simulink model "vmr_rwd_fix_leftarm"  (R2015a)
settings: Solver=ode4  SolverMode=MultiTasking  StartTime=0.0  StopTime=inf  FixedStep=BKIN_STEP_TIME  RelTol=1e-3
StartFcn:
  |  warndlg('Dexterit-E models cannot run under simulation. Please compile your model and run it from within Dexterit-E.');set_param(bdroot,'SimulationCommand','stop')
model workspace (MAT data in the model file):
  BKIN_STEP_TIME = 0.00025
  col_x = 1
  col_y = 2
  E_TARGET_ON = 3
  LOGICAL_RADIUS = 4
  START_TARGET_COL = 1
  END_TARGET_COL = 2
  ROTATION_CENTER = 3
  MAXREACHTIME_COL = 5
  ROTATION_TYPE = 7
  ROTATION = 8
  DELAY_POSTTRIAL_COL = 6
  E_STAY_CENTER = 2
  VISUAL_RADIUS = 3
  COLOR = 5
  K_SCORETEXT_ROW = 1
  LABEL_HEIGHT = 8
  HITCOLOR = 6
  E_HIT_TARGET = 5
  E_MISS_TARGET = 9
  K_REWARD_VAL = 2
  K_TONE_HIT_DURATION = 4
  K_TONE_HIT_FREQUENCY = 5
  K_VIS_RAD = 6
  E_REWARD = 6
  WAIT_AT_START_COL = 4
  LABEL = 7
  K_RETURN_RING_ROW = 7
  STROKE_WIDTH = 9
  STROKE_COLOR = 10
  K_SCORE_TIME = 8
  HAND_VIS_COL = 9
  CLAMP_COL = 10
  DO_REWARD_COL = 11
  K_TONE_NEUTRAL_DURATION = 10
  K_TONE_NEUTRAL_FREQUENCY = 11
  E_NEUTRAL_FDBK = 10
  E_SHOW_SCORE = 17
  DISPLAY_TRIAL_COL = 12
  K_INSTRUCT_TIME = 9
  E_SHOW_INSTRUCT = 18
  INSTRUCT_PAUSE_BTN = 2
  K_LEFTHAND_TGT = 12
  K_ROBOT_RAMP_TIME = 14
  K_ROBOT_MOVE_TIME = 15
  K_FIX_LEFTHAND = 13
  BKIN_KINEMATIC_FRAME_SIZE = 400
  E_NO_EVENT = 0
  K_UNUSED = 3
  ROTATED_COLOR = 11
undefined symbols (not defined in the file or in its folder): slselsubs
libraries: Video x9, slrtlib x7, General x3, KINARM_general x2, KINARM_loads x2, simulink x1, xpcnilib x1
(part 2 of 2)

== stateflow chart vmr_rwd_fix_leftarm/Trial_Control ==
  settings: sampleTime=0.001
  state MoveHandAway/
    robot_enable_controller = 1;
    tickCount = TaskwideParams[K_ROBOT_RAMP_TIME];
    tickCount += TaskwideParams[K_ROBOT_MOVE_TIME];
  state Initialize/
    // Turn off both targets, set hand_feedback on
    targetA_state=0;
    targetB_state=0;
    reward_state = 0;
    score = 0;
    rotation_on = 0;
    handvis_state = 1;
    reward_type = 0;
    instruct_num = 0;
    fdbk_text = 0;
    robot_enable_controller = 0;
  state InitStartTarget/
    // Turn on first target, wait until hand-is-in-target
    targetA_row = Trial_Protocol[START_TARGET_COL];
    targetA_state=1;
    handvis_state = 1;
    rotation_on = 0;
  state Main_Trial
    state StartTargetOn/
      // Turn on first target, wait until hand-is-in-target
      targetA_row = Trial_Protocol[START_TARGET_COL];
      targetA_state=1;
      handvis_state = 1;
      rotation_on = 0;
      logging_enable = 1;
      reward_type = Trial_Protocol[DO_REWARD_COL];
      tone = 0;
    state StayAtFirstTarget/
      // change the first target state (e.g. colour), log an event, wait for specified period of time.  Hand must STAY in target for specified time.
      event_code=E_STAY_CENTER;
      tickCount =Trial_Protocol[WAIT_AT_START_COL];
    state WaitForSound/
    state Show2ndTarget/
      // Turn on second target, log an event, wait until hand-is-in-target or wait for specified delay
      event_code=E_TARGET_ON;
      targetB_row = Trial_Protocol[END_TARGET_COL];
      targetB_state= 1 + 2*double(rotation_on > 0 || do_clamp > 0);
      tickCount =Trial_Protocol[MAXREACHTIME_COL];
      tick = 0;
      dist  = TargetDistance[START_TARGET_COL][END_TARGET_COL];
      during:
      on e_clk: tick++;
    state Hit2ndTarget/
      // change the 2nd target's state, log an event, wait for the rest of the trial to end
      event_code=E_HIT_TARGET;
    state Miss2ndTarget/
      //if hand exceeds target ring, trial is over
      event_code = E_MISS_TARGET;
      targetB_state = 0;
      reward_state = 0;
      handvis_state = 0;
      rotation_on = 0;
      during:
      on e_clk: tick++;
    state TooSlowState/
      fdbk_text = -1;  //"too slow"
      targetA_state = 2;
      rotation_on = 0;
      handvis_state = 0;
      //fdbk_text = 1; //"too fast"
    state DoReward/
      event_code = E_REWARD;
      targetB_state=2;
      reward_state=1;
      reward = TaskwideParams[K_REWARD_VAL];
      score += reward;
      fdbk_text = 0;
      tone = 1;
      handvis_state = 0;
      rotation_on = 0;
      during:
      on e_clk: tick++;
    state NeutralReward/
      event_code = E_NEUTRAL_FDBK;
      //do this state if we are in a clamped or aftereffect trial to indicate end of trial
      handvis_state = 0;
      reward_state = 0;
      fdbk_text = 0;
      rotation_on = 0;
      tone = 2;
      //do nothing
      during:
      on e_clk: tick++;
    state NoReward/
      handvis_state = 0;
      fdbk_text = 0;
      rotation_on = 0;
      //do nothing
      during:
      on e_clk: tick++;
    state EndOfTrial/
      // Wait for a specified period of time,
      targetB_state = 0;
      handvis_state = 2;
      do_clamp = 0;
      rotation_on = 0;
    StartTargetOn -> StayAtFirstTarget : [HandInTarget[targetA_row]==1]
    StayAtFirstTarget -> StartTargetOn [order 2] : [HandInTarget[targetA_row]==0]
    StayAtFirstTarget -> WaitForSound [order 1] : after(tickCount, e_clk)/
        | rotation_on = Trial_Protocol[ROTATION_TYPE];
        | handvis_state = Trial_Protocol[HAND_VIS_COL];
        | do_clamp = Trial_Protocol[CLAMP_COL];
        | e_ApplyNewRotation
        | // apply the new rotation amount now (i.e. wait until hand is in the start target so that
        | // the hand feedback doesn't jump when a new rotation is applied)
    WaitForSound -> Show2ndTarget : [soundON == 0]
    Show2ndTarget -> TooSlowState [order 1] : [tick >= tickCount]
        | //max trial duration specified by tickCount
    Show2ndTarget -> Miss2ndTarget [order 2] : [DistFromTarget[targetA_row] >= dist]
    Show2ndTarget -> Hit2ndTarget [order 3] : [HandInTarget[targetB_row]==1]
    Hit2ndTarget -> DoReward [order 3] : [reward_type == 1]
        | //do the reward
    Hit2ndTarget -> NoReward [order 2] : [reward_type == 0]
        | //no reward
    Hit2ndTarget -> NeutralReward [order 1] : [reward_type == 2]
        | //neutral feedback tone
    Miss2ndTarget -> NeutralReward [order 2] : [reward_type == 2]
        | //neutral feedback tone
    TooSlowState -> EndOfTrial
    Miss2ndTarget -> EndOfTrial [order 1] : //after(tickCount, e_clk)
        | [reward_type != 2 && tick >= tickCount]
    NoReward -> EndOfTrial : //after(tickCount, e_clk)
        | [tick >= tickCount]
    NeutralReward -> EndOfTrial : //after(tickCount, e_clk)
        | [tick >= tickCount]
    DoReward -> EndOfTrial : //after(tickCount, e_clk)
        | [tick >= tickCount]
  state Ending/
    //end the special "show score" state
    e_Trial_End;
  state EndInstructPause/
    instruct_num = 0;
    handvis_state = 1;
    targetA_state = 1;
    tickCount = 800;
  state ReturnToStart1/
    targetA_state=1;
    handvis_state = 1;
    reward_state = 0;
    instruct_num = 0;
  state InstructWaitState/
    //"pause" here until the button has been clicked
  state ShowScoreState/
    event_code = E_SHOW_SCORE;
    targetA_state = 0;
    targetB_state = 0;
    handvis_state = 1;
    reward_state = 2;
    tickCount = TaskwideParams[K_SCORE_TIME];
  state ShowInstructState/
    event_code = E_SHOW_INSTRUCT;
    targetA_state = 0;
    targetB_state = 0;
    handvis_state = 0;
    reward_state = 0;
    instruct_num = Trial_Protocol[DISPLAY_TRIAL_COL];
    tickCount = TaskwideParams[K_INSTRUCT_TIME];
  state Inter_Trial_State/
    // send e_Trial_End event
    e_Trial_End;
    // turn off both targets
    // stop data logging
    event_code=0;
    targetA_state=1; //don't shut off
    targetB_state=0;
    //logging_enable = 0;
    rotation_on = 0;
    fdbk_text = 0;
  state ReturnToStart/
    //targetA_state=1;
    handvis_state = 1;
    reward_state = 0;
    instruct_num = 0;
    tickCount =50;
  state Inter_Trial_Hold/
    //temporarily hold here until the hand gets close to the target
    tickCount = Trial_Protocol[DELAY_POSTTRIAL_COL];
  InitStartTarget -> MoveHandAway [order 1] : [HandInTarget[targetA_row]==1 && TaskwideParams[K_FIX_LEFTHAND] == 1]
      | //if we want to hold the left hand, enable the robot
  (default) -> Initialize
  MoveHandAway -> (junction 112) : after(tickCount,e_clk)
  Initialize -> InitStartTarget : after(1,e_clk)
  InitStartTarget -> (junction 112) [order 2] : [TaskwideParams[K_FIX_LEFTHAND] ~= 1]
      | //if we aren't going to enable the robot
  (junction 112) -> StartTargetOn [order 1] : [Trial_Protocol[DISPLAY_TRIAL_COL] <= 0]
      | //the first trial is a target trial
  (junction 112) -> ShowInstructState [order 2] : //the first trial is an instruction trial
      | [Trial_Protocol[DISPLAY_TRIAL_COL] > 0]
  ReturnToStart1 -> StartTargetOn : after(1, e_clk)
  Ending -> EndInstructPause : after(1,e_clk)/
      | //continue if a regular trial comes after!
  InstructWaitState -> Ending : e_cntl_btn/
      | event_code = 22;
  ShowScoreState -> Ending : after(tickCount,e_clk)
  EndInstructPause -> ReturnToStart1 : after(tickCount,e_clk)
  ShowInstructState -> InstructWaitState
  (junction 74) -> ReturnToStart1 [order 1] : [Trial_Protocol[DISPLAY_TRIAL_COL] == 0]
  (junction 74) -> ShowScoreState [order 2] : [Trial_Protocol[DISPLAY_TRIAL_COL] == -1]
  (junction 74) -> ShowInstructState [order 3] : [Trial_Protocol[DISPLAY_TRIAL_COL] > 0]
  Inter_Trial_State -> (junction 74) : after(1,e_clk)
  Main_Trial -> Inter_Trial_State : e_ExitTrialNow/
      | // if e_ExitTrialNow event occurs...
      | tickCount=1;
  ReturnToStart -> Inter_Trial_State : after(tickCount,e_clk)
  Inter_Trial_Hold -> ReturnToStart : [ DistFromTarget[targetA_row] <= TaskwideParams[K_VIS_RAD] && after(tickCount,e_clk) ]
      | //if the hand is close to the start, turn vision of the hand back on
  EndOfTrial -> Inter_Trial_Hold
  data: logging_enable output boolean; event_code output double; Trial_Protocol input double; targetA_row output [1..32]; targetA_state output double; targetB_row output double; targetB_state output double; tickCount local double; reward_state output double; score output int32; reward output int32; fdbk_text output int32; instruct_num output double; tone output double; TaskwideParams input double; HandInTarget input double; DistFromTarget input double; TargetDistance input double; reward_type local double; rotation_on output double; dist local double; tick local double; handvis_state output double; do_clamp output double; E_SHOW_INSTRUCT parameter; robot_enable_controller output boolean; soundON input double size=1
  data targetA_row settings: description=index of the row currently being used in the TargetTable
  events: e_ApplyNewRotation output EITHER_EDGE_EVENT; e_clk input RISING_EDGE_EVENT; e_ExitTrialNow input EITHER_EDGE_EVENT; e_Trial_End output EITHER_EDGE_EVENT; e_cntl_btn input EITHER_EDGE_EVENT

== matlab function vmr_rwd_fix_leftarm/Visual_Rotation/Triggered Subsystem/Embedded MATLAB Function ==
  settings: fimath=|
      | fimath(...
      | 'RoundMode', 'floor',...
      | 'OverflowMode', 'wrap',...
      | 'ProductMode', 'KeepLSB', 'ProductWordLength', 32,...
      | 'SumMode', 'KeepLSB', 'SumWordLength', 32,...
      | 'CastBeforeSum', false)
  data: rotate_on input; rotation output; Trial_Protocol input
function rotation   = Calculate_Desired_Rotation(rotate_on,Trial_Protocol)
% This block supports an embeddable subset of the MATLAB language.
% See the help menu for details. 

%This block was modified by IEB, Sept 24, 2008
%It updates the desired amount of rotation

% NOTE ALL ROTATIONS ARE CURRENTLY IN DEGREES IN THE FUNCTION

% create a persistent variable to remember the rotation amount from one time-step to the next
persistent rotation_memory

if isempty(rotation_memory),            rotation_memory = 0;										end

% where to look in the TP table for these parameters
rotate_type_COL = 7;
rotation_amount_COL = 8;

rotate_type = Trial_Protocol(rotate_type_COL);
rotation_amount = Trial_Protocol(rotation_amount_COL);

if rotate_type == 0 || rotate_on == 0
	%set the rotation = 0
	rotation = 0;
elseif rotate_type ==1 && rotate_on > 0
	%set the rotation = specified amount
	rotation = rotation_amount;
elseif rotate_type == 2 && rotate_on > 0
	%set the rotation to change by specified amount
	rotation = rotation_memory + rotation_amount;
else
	%do nothing
	rotation = rotation_memory;
end

% save the rotation amount for the next time-step
rotation_memory = rotation;

== matlab function vmr_rwd_fix_leftarm/Visual_Rotation/Embedded MATLAB Function ==
  settings: fimath=|
      | fimath(...
      | 'RoundMode', 'floor',...
      | 'OverflowMode', 'wrap',...
      | 'ProductMode', 'KeepLSB', 'ProductWordLength', 32,...
      | 'SumMode', 'KeepLSB', 'SumWordLength', 32,...
      | 'CastBeforeSum', false)
  data: CursorPos output; rotation input; TGT_VCODES_IN input; VCODES_IN input; feedback_state input; VCODES output
function [CursorPos,VCODES]  = Rotation(rotation, TGT_VCODES_IN,VCODES_IN,feedback_state) %Trial_Protocol, Target_Table,
% This block supports an embeddable subset of the MATLAB language.
% See the help menu for details. 

%This block was modified by IEB, Sept 24, 2008
%It rotates the cursor position around a location specified as a target in the Trial_Protocol.

% VCODEs are length VCODE_LENGTH.
% All dimensions are units of (m).
% VCODE index definition: 1-5 as the same for all target types
% 1 - Target type
%		1=circle
%		2=ellipse
%       3=rectangle
%		4=line
%       5=triangle
%		6 and higher - not implemented yet
% 2 - status
%		0=off
%		1=on
% 3 - x position (m)
% 4 - y position (m)

% column in target table to find the target to rotation about
rotation_center_COL = 3;

%rotation_center_target = Trial_Protocol(rotation_center_COL);
%x_center = Target_Table(rotation_center_target, 1) * 0.01;		%convert to meters
%y_center = Target_Table(rotation_center_target, 2) * 0.01;		%convert to meters
x_center = TGT_VCODES_IN(3);
y_center = TGT_VCODES_IN(4);

rotation = rotation*pi/180;		%convert desired rotation from degrees to radians

VCODES = VCODES_IN;
CursorPos = VCODES(1:2,3:4);
T = [x_center, y_center; x_center, y_center];                       %translation matrix
R = [cos(rotation) -sin(rotation); sin(rotation) cos(rotation)];	%rotation matrix

CursorPos = CursorPos - T;				%translate
CursorPos = (R*CursorPos')';			%rotate
CursorPos = CursorPos + T;				%re-translate

VCODES(1:2,3:4) = CursorPos;			%apply updated positions back into the VCODEs		

VCODES(1:2,1) = VCODES(1:2,1) & feedback_state;

== matlab function vmr_rwd_fix_leftarm/KINARM_HandFeedbackInTarget/Embedded MATLAB InsideTarget ==
  settings: fimath=|
      | fimath(...
      | 'RoundMode', 'floor',...
      | 'OverflowMode', 'wrap',...
      | 'ProductMode', 'KeepLSB', 'ProductWordLength', 32,...
      | 'SumMode', 'KeepLSB', 'SumWordLength', 32,...
      | 'CastBeforeSum', false)
  data: handpos input size=2; target_type input; attribcol input; num_targets input; intarget output; Target_Table input
function intarget = FIsInsideTarget(handpos, target_type, attribcol, num_targets, Target_Table)
% all dimensions in m, rad
% arguments:
% handpos: x,y positions of center of target
% attribcol: columns in target table specifying target attributes.  
% Specific to Target_Type
%	circle:
%	[X0,Y0,r...,rn] where:
%	X0,Y0 : centre of circle
%	r : logical radius of circle (i.e. radius used to determine 'in' or 'out' of target)
%	rn: logical radius of other targets (e.g. 2nd, 3rd) also specified in target row.
%   Up to 4 targets can be specified in a row
% ellipse:
%	[X0,Y0,a,b,t...,an, bn, tn] where:
%	X0,Y0 : centre of ellipse
%	a,b : major, minor radii of ellipse
%	t : rotation of ellipse in degrees
%	an,bn : major, minor radii of ellipse of other targets (e.g. 2nd, 3rd) also specified in target row
%	tn : rotation of ellipse in degrees of other targets (e.g. 2nd, 3rd) also specified in target row
%   Up to 4 targets can be specified in a row


target_col_x=1;
target_col_y=2;

x=handpos(1);
y=handpos(2);

intarget = zeros(size(Target_Table,1),4);

X0 = Target_Table(:,target_col_x)*0.01;			%Target Table sizes in cm in v1.4
Y0 = Target_Table(:,target_col_y)*0.01;			%Target Table sizes in cm in v1.4

deltax=x-X0;
deltay=y-Y0;

INT_MAX=2^32-1;

if target_type==1			%circle
	for target=1:num_targets
		r = Target_Table(:,attribcol(target))*0.01;			%Target Table sizes in cm in v1.4
		% simple euclidean distance
		distance2 = deltax.^2 + deltay.^2;					%distance2 is the square of the distance
	    intarget(:,target) = (distance2 <= r.^2);
	end
elseif target_type==2		%ellipse
	for target=1:num_targets
	    a = Target_Table(:,attribcol(target*3-2))*0.01;			%Target Table sizes in cm in v1.4
	    b = Target_Table(:,attribcol(target*3-1))*0.01;			%Target Table sizes in cm in v1.4	
	    t = Target_Table(:,attribcol(target*3))*(pi / 180.0);	%Target Table angles in degrees in v1.4
		sint=sin(t);
		cost=cos(t);
		xrotate=deltax.*cost+deltay.*sint;		%location of x point in ellipse's coordinate frame
		yrotate=-deltax.*sint+deltay.*cost;		%location of y point in ellipse's coordinate frame
		m=yrotate./xrotate;						%slope of line between the (x,y) to (x0,y0) in ellipse's coordinate frame
		y2sq=1./(1./(m.*a).^2+1./b.^2);			%y2sq is y2^2, where y2 is the intersection of the ellipse and the (x,y) to (x0,y0) line
	    intarget(:,target) = (yrotate.^2 <= y2sq);
    end
elseif target_type==3       %rectangle
    for target=1:num_targets
        w = Target_Table(:,attribcol(target*3-2))*0.01;  %width (sizes in cm in v1.4)
        h = Target_Table(:,attribcol(target*3-1))*0.01;  %height (sizes in cm in v1.4)
        
        if attribcol(target*3) > 0
            t = Target_Table(:,attribcol(target*3))*(pi / 180.0);  %angle (angles in degrees in v1.4)
        else
            t = zeros(size(Target_Table, 1), 1);
        end

        sint=sin(t);
        cost=cos(t);

        xrotate=deltax.*cost + deltay.*sint;   %location of x point in rectangle's coordinate frame
        yrotate=-deltax.*sint + deltay.*cost;  %location of y point in rectangle's coordinate frame

        intarget(:,target) = abs(xrotate) <= w/2 & abs(yrotate) <= h/2;
    end
elseif target_type==4       %line
    for target=1:num_targets
        % treat the line like a rectangle of height h and width w
        % determine height (stroke width) in the same fashion as in Show_Target
        if attribcol(target*3-2) == 0                     %0 column index means stroke width of 0
            h = zeros(size(Target_Table, 1), 1);
        elseif attribcol(target*3-2) < 0                  %-ve column index means stroke width of 1mm
            h = ones(size(Target_Table, 1), 1) .* 0.001;
        else
            h = Target_Table(:,attribcol(target*3-2)) * 0.01;  %target table contains width in cm
        end
        
        ex = Target_Table(:,attribcol(target*3-1))*0.01;  %endpoint in x relative to start point (cm)
        ey = Target_Table(:,attribcol(target*3))*0.01;    %endpoint in y relative to start point (cm)
        
        w = sqrt(ex.^2 + ey.^2);                          %width (cm)
        
        % determine the vector from the line's midpoint to the hand position
        handx = deltax - ex/2;
        handy = deltay - ey/2;
        
        t = atan2(ey, ex);                                %calculate angle of the line (rads)
        sint = sin(t);
        cost = cos(t);
        
        xrotate = handx.*cost + handy.*sint;   %location of x point in rectangle's coordinate frame
        yrotate = -handx.*sint + handy.*cost;  %location of y point in rectangle's coordinate frame
 
        intarget(:,target) = abs(xrotate) <= w/2 & abs(yrotate) <= h/2;
    end
elseif target_type==5  % triangle
    for target=1:num_targets
        w = Target_Table(:,attribcol(target*4-3))*0.01;         %length (sizes in cm in v1.4)
        
        % If a height column of 0 is specified, make the triangle equilateral. Otherwise, use the
        % values for height and peak offset from the target table.
        if attribcol(target*4-2) > 0
            h = Target_Table(:,attribcol(target*4-2))*0.01;  %height (sizes in cm in v1.4)
            p = Target_Table(:,attribcol(target*4-1))*0.01;  %peak offset (sizes in cm in v1.4)
        else
            h = w.*sin(pi/3.0);
            p = zeros(size(Target_Table, 1), 1);
        end
        
        if attribcol(target*4) > 0
            t = Target_Table(:,attribcol(target*4))*(pi / 180.0);  %angle (angles in degrees in v1.4)
        else
            t = zeros(size(Target_Table, 1), 1);
        end
        
        sint = sin(t);
        cost = cos(t);
        
        xrotate = deltax.*cost + deltay.*sint;   %location of x point in triangle's coordinate frame
        yrotate = -deltax.*sint + deltay.*cost;  %location of y point in triangle's coordinate frame
        
        % Begin to find centroid of triangle relative to the point on the base beneath the peak. "Left vertex" 
        % refers to the vertex at the left end of the base, and "right vertex" to the vertex at the right end.
        n = w./2.0 + p;  % distance along base from left vertex to peak
        m = w./2.0 - p;  % distance along base from peak to right vertex

        alpha = atan2(h, n);  % angle between base and line from left vertex to peak
        beta = atan2(h, m);   % angle between base and line from right vertex to peak
        
        length1 = sqrt(h.*h + n.*n) ./ 2.0;  % half length of line from left vertex to peak
        length2 = sqrt(h.*h + m.*m) ./ 2.0;  % half length of line from right vertex to peak

        % Determine slope of line from left vertex to midpoint of line from right vertex to peak.
        slope1 = ones(size(Target_Table, 1), 1) .* INT_MAX;
        
        for i=1:size(Target_Table, 1)
            if abs(w(i) - length2(i)*cos(beta(i))) > 0.0
                slope1(i) = length2(i)*sin(beta(i)) / (w(i) - length2(i)*cos(beta(i)));
            end
        end

        % Determine slope of line from right vertex to midpoint of line from left vertex to peak.
        slope2 = ones(size(Target_Table, 1), 1) .* INT_MAX;

        for i=1:size(Target_Table, 1)
            if abs(w(i) - length1(i)*cos(alpha(i))) > 0.0
                slope2(i) = -length1(i)*sin(alpha(i)) / (w(i) - length1(i)*cos(alpha(i)));
            end
        end

        % Calculate centroid position.
        centroid_x = -(m.*slope2 + n.*slope1) ./ (slope1 - slope2);
        centroid_y = slope1.*(centroid_x + n);

        % Test if the point is under the left side of the peak.
        is_under_left = false(size(Target_Table, 1), 1);

        for i=1:size(Target_Table, 1)
            if n(i) >= 0
                is_under_left(i) = (h(i) + (h(i)/n(i)) * (xrotate(i) + centroid_x(i))) >= (yrotate(i) + centroid_y(i));
            else
                is_under_left(i) = (h(i) + (h(i)/n(i)) * (xrotate(i) + centroid_x(i))) <= (yrotate(i) + centroid_y(i));
            end
        end
        
        % Test if the point is under the right side of the peak.
        is_under_right = false(size(Target_Table, 1), 1);

        for i=1:size(Target_Table, 1)
            if m(i) >= 0
                is_under_right(i) = (h(i) - (h(i)/m(i)) * (xrotate(i) + centroid_x(i))) >= (yrotate(i) + centroid_y(i));
            else
                is_under_right(i) = (h(i) - (h(i)/m(i)) * (xrotate(i) + centroid_x(i))) <= (yrotate(i) + centroid_y(i));
            end
        end
        
        intarget(:,target) = is_under_right & ...            %under right side of peak
                             is_under_left & ...             %under left side of peak
                             (yrotate + centroid_y) >= 0.0;  %above base
    end
end

== matlab function vmr_rwd_fix_leftarm/KINARM_HandFeedbackInTarget/Embedded MATLAB WhichHand ==
  settings: fimath=|
      | fimath(...
      | 'RoundMode', 'floor',...
      | 'OverflowMode', 'wrap',...
      | 'ProductMode', 'KeepLSB', 'ProductWordLength', 32,...
      | 'SumMode', 'KeepLSB', 'SumWordLength', 32,...
      | 'CastBeforeSum', false)
  data: use_dominant_hand input; dominant_hand input; hand output; cursor output
function [hand, cursor] = WhichHand(use_dominant_hand, dominant_hand)

if use_dominant_hand==1				%use the dominant hand
	hand=dominant_hand;		
	cursor = 1;
else
	hand=3-dominant_hand;			%use the non-dominant hand. i.e. if dominant_hand=2, hand=1 and vice-versa
	cursor = 2;
end

== matlab function vmr_rwd_fix_leftarm/DisplayText/MATLAB Function ==
  data: VCODE input; score input; VCODE_mod output; fdbk_text input; start_tgt_VCODE input
function VCODE_mod = fcn(VCODE,score,fdbk_text,start_tgt_VCODE)


VCODE_mod = VCODE;

if (fdbk_text == 0)  %if this is zero, show the score
       
    
    %score is in cents. potentially need to convert to dollars
    
    if (score < 10)
        text1 = 'You earned ';
        text2 = ' cents!';
        
        textout = [text1 int2char(int32(score)) text2];
        
    elseif (score < 100) %score < $1
        text1 = 'You earned ';
        text2 = ' cents!';
        
        n1 = int32(floor(double(score)/10));  %we need to cast score to a double otherwise the arithmetic is wrong!
        n2 = score - n1*10;
        
        textout = [text1 int2char(int32(n1)) int2char(int32(n2)) text2];
        
    else %score > $1, convert to dollars to keep the score readable
        text1 = 'You earned $';
        text2 = '.';
        text3 = '!';
        
        dollars = int32(floor(double(score)/100));
        if (dollars >= 10) %double digit dollar value
            n1d = int32(floor(double(dollars)/10));
            n2d = dollars - n1d*10;
            textdollars = [int2char(int32(n1d)) int2char(int32(n2d))];
        else %single digit
            textdollars = int2char(int32(dollars));
        end
        
        cents = score-dollars*100;
        if (cents < 10)
            textcents = ['0' int2char(int32(cents))];
        else
            n1 = int32(floor(double(cents)/10));
            n2 = round(cents - n1*10);
            textcents = [int2char(int32(n1)) int2char(int32(n2))];
        end
        
        textout = [text1 textdollars text2 textcents text3];
        
    end
    
elseif (fdbk_text == 1) 
    %print "too fast"
    textout = 'Too Fast!';
    
    
elseif (fdbk_text == -1) 
    %print "too slow"
    
    textout = 'Too Slow!';
else
    textout = '';
    
end
    

%the first character is VCODE(15)
%need to translate text into ascii:
textnum = double(textout); %this quickly casts each char into a number

%make sure we won't overflow the VCODE: no more than 50 chars! we will
%clip off anything that overflows.
VCODE_mod(1,15:min([15+length(textout),64])) = textnum(1:min([length(textnum),50])); %write out as many the characters as possible into the VCODE
VCODE_mod(1,min([15+length(textout)+1,64])) = 0;  %terminate the string!

VCODE_mod(1,3) = start_tgt_VCODE(1,3);



function s = int2char(n)

n = mod(n,10); %make sure we only have 1 digit or we will get a weird character!

s = char(n+int32('0')); %// add the character

== matlab function vmr_rwd_fix_leftarm/KINARM_DistanceBetweenTargets/Embedded MATLAB InsideTarget ==
  settings: fimath=|
      | fimath(...
      | 'RoundMode', 'floor',...
      | 'OverflowMode', 'wrap',...
      | 'ProductMode', 'KeepLSB', 'ProductWordLength', 32,...
      | 'SumMode', 'KeepLSB', 'SumWordLength', 32,...
      | 'CastBeforeSum', false)
  data: distance output; Target_Table input
function distance = Distance(Target_Table)
% all dimensions in m, rad
% arguments:
% handpos: x,y positions of center of target

target_col_x=1;
target_col_y=2;

X0 = Target_Table(:,target_col_x)*0.01;			%Target Table sizes in cm in v1.4
Y0 = Target_Table(:,target_col_y)*0.01;			%Target Table sizes in cm in v1.4

Xdif = repmat(X0,1,length(X0))-repmat(X0',length(X0),1);
Ydif = repmat(Y0,1,length(Y0))-repmat(Y0',length(Y0),1);

distance = sqrt(Xdif.^2 + Ydif.^2);

== matlab function vmr_rwd_fix_leftarm/Visual_Rotation/MATLAB Function ==
  data: TGTVCODE_IN input; VCODE_IN input; VCODE output; dist_from_target input; tgt_row input
function VCODE = ReturnRing(TGTVCODE_IN,VCODE_IN,dist_from_target,tgt_row)
%#codegen

VCODE = [VCODE_IN; VCODE_IN];  %duplicate this to make it a 2x70 matrix to match
Start_Tgt_VCODE = TGTVCODE_IN(1,:);

VCODE(1,3:4) = Start_Tgt_VCODE(3:4);
VCODE(2,3:4) = Start_Tgt_VCODE(3:4);

VCODE(1:2,10) = dist_from_target(tgt_row);  %set the radius to be the distance from the start position

VCODE(2,2) = 0;  %disable the duplicate

== matlab function vmr_rwd_fix_leftarm/Visual_Rotation/Embedded MATLAB Function1 ==
  settings: fimath=|
      | fimath(...
      | 'RoundMode', 'floor',...
      | 'OverflowMode', 'wrap',...
      | 'ProductMode', 'KeepLSB', 'ProductWordLength', 32,...
      | 'SumMode', 'KeepLSB', 'SumWordLength', 32,...
      | 'CastBeforeSum', false)
  data: Trial_Protocol input; VCODES output; TGTVCODES_IN input; VCODES_IN input; CursorPos output; dist_from_target input; feedback_state input
function [VCODES, CursorPos]  = Clamp(Trial_Protocol,TGTVCODES_IN,VCODES_IN,dist_from_target,feedback_state) %Trial_Protocol, Target_Table
% This block supports an embeddable subset of the MATLAB language.
% See the help menu for details. 

%This block clamps the cursor position along the vector between the start
%and reach targets

% VCODEs are length VCODE_LENGTH.
% All dimensions are units of (m).
% VCODE index definition: 1-5 as the same for all target types
% 1 - Target type
%		1=circle
%		2=ellipse
%       3=rectangle
%		4=line
%       5=triangle
%		6 and higher - not implemented yet
% 2 - status
%		0=off
%		1=on
% 3 - x position (m)
% 4 - y position (m)

start_tgt_COL = 1; %column of the start target in the Trial Protocol Table
reach_tgt_COL = 2; %column of the start target in the Trial Protocol Table

%start_target = Trial_Protocol(start_tgt_COL);
%start_target_x = Target_Table(start_target, 1) * 0.01;		%convert to meters
%start_target_y = Target_Table(start_target, 2) * 0.01;		%convert to meters
start_target_x = TGTVCODES_IN(1,3);
start_target_y = TGTVCODES_IN(1,4);

%reach_target = Trial_Protocol(reach_tgt_COL);
%reach_target_x = Target_Table(reach_target, 1) * 0.01;		%convert to meters
%reach_target_y = Target_Table(reach_target, 2) * 0.01;		%convert to meters
reach_target_x = TGTVCODES_IN(2,3);
reach_target_y = TGTVCODES_IN(2,4);
tgt_vec = [reach_target_x - start_target_x,reach_target_y - start_target_y];

VCODES = VCODES_IN;
CursorPos = VCODES(1:2,3:4);


%get the absolute distance of the hand from the start target, in meters
starttgt = Trial_Protocol(start_tgt_COL);
hand_dist = abs(dist_from_target(starttgt));

%get the distance of the reach target from the start target, in meters
tgt_dist = sqrt( sum(tgt_vec.^2) );

%project the hand distance along the start-reach vector
u = tgt_vec*(hand_dist/tgt_dist);
CursorPos(:,1) = start_target_x + u(1);
CursorPos(:,2) = start_target_y + u(2);

VCODES(1,3:4) = CursorPos(1,:);
VCODES(2,3:4) = CursorPos(2,:);
%VCODES(1:2,3:4) = CursorPos;			%apply updated positions back into the VCODEs		



VCODES(1:2,1) = VCODES(1:2,1) & feedback_state;

== matlab function vmr_rwd_fix_leftarm/Visual_Rotation/MATLAB Function1 ==
  data: cursstate output; fbswitch output; fdbkstate input; ringstate output
function [cursstate,fbswitch,ringstate] = setvis(fdbkstate)
%#codegen


%if feedback_state is not 2 (the ring), pass it to modulate the cursor enable
if (fdbkstate < 1.5)
    cursstate = fdbkstate;
    ringstate = 0;
else %if feedback_state is 2 (the ring), enable the ring and disable the cursor
    cursstate = 0;
    ringstate = 1;
end

%set the switch flag appropriately
if (fdbkstate < 1.5)  %if the feedback_state is 0 or 1, switch to input 1 (cursor)
    fbswitch = 1;
else %if the feedback_state is 2, switch to input 3 (the ring)
    fbswitch = 0;
end

== stateflow chart vmr_rwd_fix_leftarm/Subsystem/Chart ==
  state EnableState/
    state AutoMoveToPos/
      //smoothly creates a trajectory to get the hand to a point eventually
      state MovingToDesiredXY/
        tickCount = TaskwideParams[K_ROBOT_MOVE_TIME];
        state = 11;
        tick = 0;
        during:
        on e_clk: tick++;
        // the trajectory velocity will have a bell shaped profile
        trajectory_shape = tick/tickCount-sin(2*pi*tick/tickCount)/(2*pi);
        virtual_pos[1] = StartPos[1] + (TgtPos[1] - StartPos[1]) * trajectory_shape;
        virtual_pos[2] = StartPos[2] + (TgtPos[2] - StartPos[2]) * trajectory_shape;
      state GetDesiredXY/
        //grab the current desired pos in case it changes
        TgtPos[1] = DesiredPos[1];
        TgtPos[2] = DesiredPos[2];
        StartPos[1] = HandPos[1];
        StartPos[2] = HandPos[2];
        updatepos = 0;
        state = 10;
      state HoldAtDesiredXY/
        //pause until something changes
        state = 12;
        updatepos = 0;
        during:
        on e_clk: updatepos = ( (abs(TgtPos[1]-DesiredPos[1]) > 0.01) || (abs(TgtPos[2]-DesiredPos[2]) > 0.01) )
      GetDesiredXY -> MovingToDesiredXY : after(1, e_clk)
      HoldAtDesiredXY -> GetDesiredXY : [updatepos == 1]
      MovingToDesiredXY -> HoldAtDesiredXY : after(tickCount, e_clk)/
  state Init/
    ramp_time = TaskwideParams[K_ROBOT_RAMP_TIME];
    scale_increment = 1/ramp_time;
    force_scale = 0;
    state = 1;
    during:
    CurHandPos[1] = HandPos[1];
    CurHandPos[2] = HandPos[2];
  state RampUp/
    //ramp up the force scale to 1
    CurHandPos[1] = HandPos[1];
    CurHandPos[2] = HandPos[2];
    virtual_pos[1] = HandPos[1];
    virtual_pos[2] = HandPos[2];
    state = 2;
    force_scale = 0;
    during:
    on e_clk: force_scale += scale_increment;
  state ResetController/
    reset_controller;
  state RampDown/
    //ramp down the force scale to 1
    CurHandPos[1] = HandPos[1];
    CurHandPos[2] = HandPos[2];
    virtual_pos[1] = CurHandPos[1];
    virtual_pos[2] = CurHandPos[2];
    state = 30
    during:
    on e_clk: force_scale -= scale_increment;
  (default) -> Init
  Init -> ResetController : //if controller becomes enabled
      | [enable_controller == 1]/
      | force_scale = 0;
  ResetController -> RampUp
  RampUp -> GetDesiredXY [order 2] : [force_scale >= 1]/
      | force_scale = 1;
  RampDown -> Init [order 2] : [force_scale <0]/
      | force_scale = 0;
  RampDown -> RampUp [order 1] : [enable_controller == 1]
      | //if the controller is enabled
  RampUp -> RampDown [order 1] : [enable_controller == 0]
      | //if the controller gets shut off
  EnableState -> RampDown : [enable_controller == 0]
  data: enable_controller input boolean; DesiredPos input; HandPos input; TaskwideParams input; force_scale output double; virtual_pos output double size=2; tickCount local double; StartPos local double size=2; TgtPos local double size=2; updatepos local boolean; CurHandPos local double size=2; ramp_time local double; scale_increment local double; tick local double; trajectory_shape local double; pi constant double =3.14159265358979; state output double
  events: e_clk input EITHER_EDGE_EVENT; reset_controller output EITHER_EDGE_EVENT

== matlab function vmr_rwd_fix_leftarm/Play Sound/Play sound over and over ==
  data: tone input; coin input; output output; neutralbeep input; soundON output
function [output,soundON] = fcn(tone,coin,neutralbeep)
%#codegen

persistent t last_tone_state
if isempty(t), t = 0; end
if isempty(last_tone_state), last_tone_state = 0; end

trigger = last_tone_state ~= tone;
if trigger > 0
    last_tone_state = tone;
end

soundON = 0;
output = 0;		% default
if t == 0 && trigger > 0
	% start the playing of the sound.
	t = t + 1;
    soundON = 1;
end

if tone == 1
    data = coin;
elseif tone == 2
    data = neutralbeep;
else 
    t = 0;
    data = 0;
end

if t > 0
	output = data(t);
	if t == length(data)
		t = 0;
        soundON = 0;
	else
		t = t + 1;
	end
end
end

== matlab function vmr_rwd_fix_leftarm/Subsystem/MATLAB Function1 ==
  data: pos input; VCODE input; VCODE_MOD output
function VCODE_MOD = get_tgtpos(pos,VCODE)
%#codegen

VCODE_MOD = VCODE;
VCODE_MOD(3) = pos(1);
VCODE_MOD(4) = pos(2);
